simulink model "mpc_regulator"  (R2020b)
settings: Solver=ode4  StartTime=0.0  StopTime=t_sim  FixedStep=T  RelTol=1e-3
values from neighbouring files (symbols this model uses):
  A = [9.5310 195.4713; 0 -5.129]    [main.m]
  B = [-7.6354; 8.0736]    [main.m]
  mpc_design = mpc_mtx_fun(mpc_par)    [main.m]
  T = 0.01    [main.m]
  x0 = [1; 1]    [main.m]
undefined symbols (not defined in the file or in its folder): Ad_sys, Bd_sys, mpc_par
settings Model: Creator=vince  LastModifiedBy=vince
settings DataIOCC: ReturnWorkspaceOutputs=off

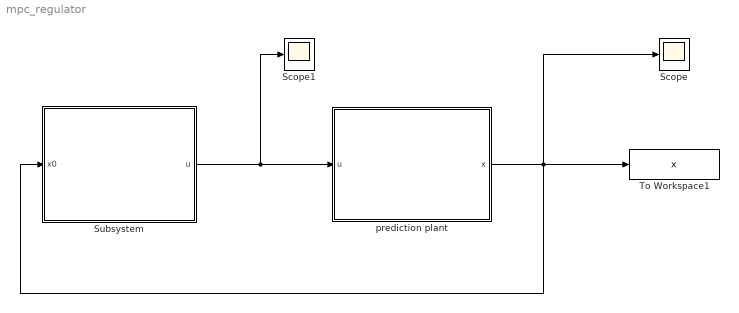
== system mpc_regulator ==
  Scope : Scope
  Scope1 : Scope
  Subsystem : Subsystem
  To Workspace1 : ToWorkspace  VariableName=x  SaveFormat=Timeseries  SampleTime=T
  prediction plant : Subsystem
  wires:
  Subsystem/1(u) -> prediction plant/1(u), Scope1/1
  prediction plant/1(x) -> Scope/1, Subsystem/1(x0), To Workspace1/1

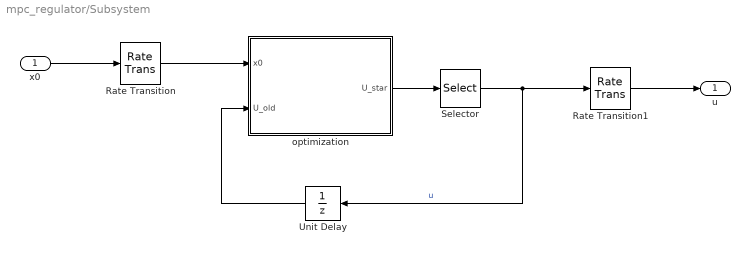
== system mpc_regulator/Subsystem ==
  x0 : Inport
  Rate Transition : RateTransition  OutPortSampleTime=mpc_par.Ts
  Rate Transition1 : RateTransition  OutPortSampleTime=T
  Selector : Selector  InputPortWidth=mpc_par.q*mpc_par.Np  IndexOptions=Index vector (dialog)  Indices=1  OutputSizes=1
  Unit Delay : UnitDelay  InitialCondition=mpc_design.U0  SampleTime=mpc_par.Ts  HasFrameUpgradeWarning=on
  optimization : MATLAB Function  TreatAsAtomicUnit=on
  u : Outport
  wires:
  optimization/1(U_star) -> Selector/1
  Selector/1 -> Unit Delay/1, Rate Transition1/1  "u"
  Rate Transition/1 -> optimization/1(x0)
  Unit Delay/1 -> optimization/2(U_old)
  x0/1 -> Rate Transition/1
  Rate Transition1/1 -> u/1

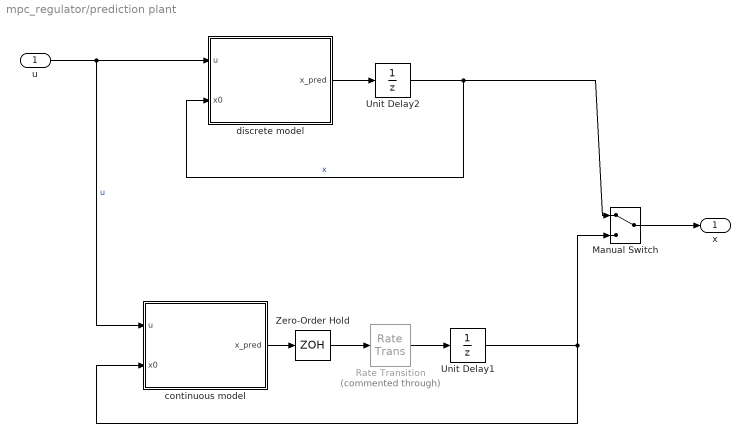
== system mpc_regulator/prediction plant ==
  u : Inport
  Manual Switch : ManualSwitch
  Rate Transition : RateTransition  Commented=through  OutPortSampleTime=T
  Unit Delay1 : UnitDelay  InitialCondition=x0  SampleTime=T  HasFrameUpgradeWarning=on
  Unit Delay2 : UnitDelay  InitialCondition=x0  SampleTime=T  HasFrameUpgradeWarning=on
  Zero-Order Hold : ZeroOrderHold  SampleTime=T
  continuous model : MATLAB Function  TreatAsAtomicUnit=on
  discrete model : MATLAB Function  TreatAsAtomicUnit=on
  x : Outport
  wires:
  discrete model/1(x_pred) -> Unit Delay2/1
  Unit Delay2/1 -> Manual Switch/1, discrete model/2(x0)  "x"
  u/1 -> discrete model/1(u), continuous model/1(u)  "u"
  Manual Switch/1 -> x/1
  Unit Delay1/1 -> continuous model/2(x0), Manual Switch/2
  Rate Transition/1 -> Unit Delay1/1
  Zero-Order Hold/1 -> Rate Transition/1
  continuous model/1(x_pred) -> Zero-Order Hold/1

== matlab function mpc_regulator/Subsystem/optimization ==
  data: U_star output; x0 input; U_old input; mpc_par parameter; mpc_design parameter
function U_star  = mpc_optimization(x0, U_old, mpc_par, mpc_design)
%% Documentation
%{
    INCOME: x, U_old
    OUTCOME: U*
%}


%% Assignment
n = mpc_par.n;
p = mpc_par.p;
q = mpc_par.q;
Np = mpc_par.Np;



%% Constraints
X_min = mpc_design.X_c(:,1);
X_max = mpc_design.X_c(:,2);
U_min = mpc_design.U_c(:,1);
U_max = mpc_design.U_c(:,2);
dU_min = mpc_design.dU_c(:,1);
dU_max = mpc_design.dU_c(:,2);



A_ineq = [-mpc_design.B_bar; mpc_design.B_bar; 
        -eye(q*Np); eye(q*Np); 
        -eye(q*Np); eye(q*Np)];
b_ineq = [-X_min+mpc_design.A_bar*x0; X_max+mpc_design.A_bar*x0;
        -U_min; U_max;
        -dU_min-U_old; dU_max+U_old];

    
%% Objective function
H = mpc_design.R_bar + mpc_design.B_bar'*mpc_design.Q_bar*mpc_design.B_bar;
H = (H+H')/2;
F = mpc_design.B_bar'*mpc_design.Q_bar*mpc_design.A_bar;
f = x0'*F';
%G = A_bar'*Q_bar*A_bar;


%% Optimization problem
% J(k) = U(k)'*H*U(k) + f'*U(k)
U_star = zeros(q*Np, 1);
coder.extrinsic('quadprog');
%options = optimoptions('quadprog', 'Algorithm', 'active-set');
U_star = quadprog(H, f, A_ineq, b_ineq, [], [], [], [], []);

== matlab function mpc_regulator/prediction plant/continuous model ==
  data: u input; x_pred output; x0 input; A parameter; B parameter
function x_pred = mpc_pred_cont(u, x0, A, B)

x = x0;
x_pred = A*x + B*u;

== matlab function mpc_regulator/prediction plant/discrete model ==
  data: u input; x_pred output; x0 input; Ad_sys parameter; Bd_sys parameter
function x_pred = mpc_pred_disc(u, x0, Ad_sys, Bd_sys)

x = x0;
x_pred = Ad_sys*x + Bd_sys*u;
